simulink model "Kalman_es1"  (R2024a)
settings: Solver=VariableStepAuto  StartTime=0.0  StopTime=10.0  RelTol=1e-3
values from neighbouring files (symbols this model uses):
  A = [-1 4;1 -5]    [TE_ES1_2023_01_09.m]
  B = [1 1]'    [TE_ES1_2023_01_09.m]
  G = eye(2)    [TE_ES1_2023_01_09.m]
  L = place(A',C1',aval_doppia)    [TE_ES1_2023_01_09.m]
  Rv = 0.01    [TE_ES1_2023_01_09.m]
  Rw = [0.1 0;0 0.01]    [TE_ES1_2023_01_09.m]
undefined symbols (not defined in the file or in its folder): C, ueq, Xo
settings Model: Creator=stefa  LastModifiedBy=stefa

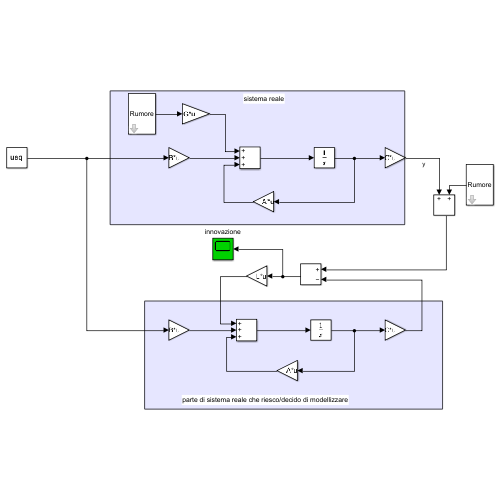
[thumbnail: Simulink's stored preview of the top-level diagram]
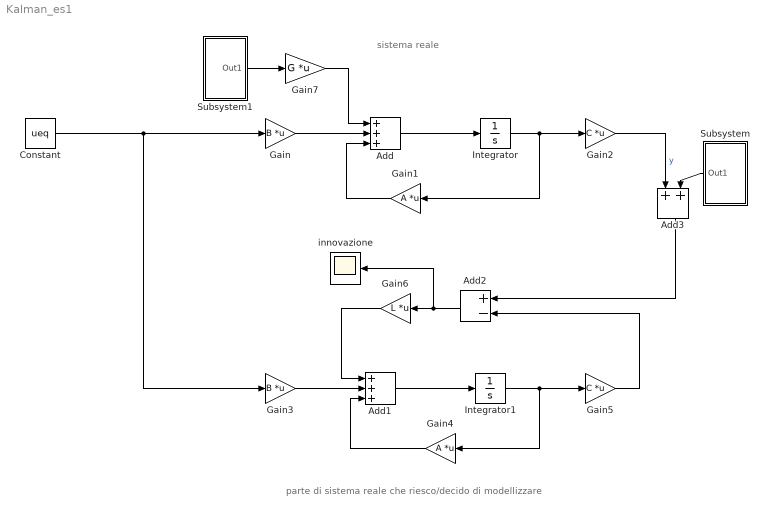
== system Kalman_es1 ==
  note: parte di sistema reale che riesco/decido di modellizzare
  note: sistema reale
  Add : Sum  Inputs=+++
  Add1 : Sum  Inputs=+++
  Add2 : Sum  Inputs=+-
  Add3 : Sum
  Constant : Constant  Value=ueq
  Gain : Gain  Gain=B  Multiplication=Matrix(K*u)
  Gain1 : Gain  Gain=A  Multiplication=Matrix(K*u)
  Gain2 : Gain  Gain=C  Multiplication=Matrix(K*u)
  Gain3 : Gain  Gain=B  Multiplication=Matrix(K*u)
  Gain4 : Gain  Gain=A  Multiplication=Matrix(K*u)
  Gain5 : Gain  Gain=C  Multiplication=Matrix(K*u)
  Gain6 : Gain  Gain=L  Multiplication=Matrix(K*u)
  Gain7 : Gain  Gain=G  Multiplication=Matrix(K*u)
  Integrator : Integrator  InitialCondition=Xo
  Integrator1 : Integrator
  Subsystem : Subsystem  mask{mat_cov=Rv}
      mask prompts: mat_cov "Covariance Matrix"
      mask Display: disp('Rumore')
  Subsystem1 : Subsystem  mask{mat_cov=Rw}
      mask prompts: mat_cov "Covariance Matrix"
      mask Display: disp('Rumore')
  innovazione : Scope
  wires:
  Gain/1 -> Add/2
  Add/1 -> Integrator/1
  Gain1/1 -> Add/3
  Integrator/1 -> Gain1/1, Gain2/1
  Integrator1/1 -> Gain4/1, Gain5/1
  Gain4/1 -> Add1/3
  Add1/1 -> Integrator1/1
  Gain3/1 -> Add1/2
  Gain6/1 -> Add1/1
  Add2/1 -> innovazione/1, Gain6/1
  Gain5/1 -> Add2/2
  Add3/1 -> Add2/1
  Subsystem/1(Out1) -> Add3/2
  Gain2/1 -> Add3/1  "y"
  Subsystem1/1(Out1) -> Gain7/1
  Gain7/1 -> Add/1
  Constant/1 -> Gain3/1, Gain/1

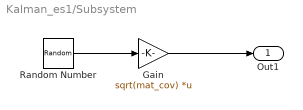
== system Kalman_es1/Subsystem ==
  Gain : Gain  Gain=sqrt(mat_cov)  Multiplication=Matrix(K*u)
  Random Number : RandomNumber  Mean=zeros(size(mat_cov,1),1)  Variance=ones(size(mat_cov,1),1)  Seed=floor([1:size(mat_cov,1)].*(abs(randn(1,size(mat_cov,1))*10)+1))  SampleTime=0.001
  Out1 : Outport  VectorParamsAs1DForOutWhenUnconnected=off
  wires:
  Random Number/1 -> Gain/1
  Gain/1 -> Out1/1

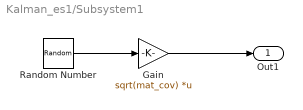
== system Kalman_es1/Subsystem1 ==
  Gain : Gain  Gain=sqrt(mat_cov)  Multiplication=Matrix(K*u)
  Random Number : RandomNumber  Mean=zeros(size(mat_cov,1),1)  Variance=ones(size(mat_cov,1),1)  Seed=floor([1:size(mat_cov,1)].*(abs(randn(1,size(mat_cov,1))*10)+1))  SampleTime=0.001
  Out1 : Outport  VectorParamsAs1DForOutWhenUnconnected=off
  wires:
  Random Number/1 -> Gain/1
  Gain/1 -> Out1/1
